simulink model "lab4_sim"  (R2022b)
settings: Solver=VariableStepAuto  StartTime=0.0  StopTime=10.0  RelTol=1e-3
values from neighbouring files (symbols this model uses):
  A = [0 0 1 0; 0 0 0 1; -(k1 + k2)/m1 k2/m1 -(c1 + c2)/m1 c2/m1; k2/m2 -k2/m2 c2/m2 -c2/m2]    [lab4.m]    (also in test.m)
  B = [(c1/m1) 0 0; 0 0 0; (k1/m1) - ((c1 + c2)*c1)/(m1*m1) (k1 + k2)/m1 k2/m1 ; (c1*c2)/(m1*m2) k2/m2 -k2/m2]    [lab4.m]    (also in test.m = [(c1/m1); 0; (k1/m1) - ((c1 + c2)*c1)/(m1*m1); (c1*c2)/(m1*m)
  C = [1 0 0 0; 0 1 0 0; 0 0 1 0; 0 0 0 1]    [lab4.m]    (also in test.m = eye(4,4))
  c1 = 100    [lab4.m]    (also in test.m)
  c2 = 2000    [lab4.m]    (also in test.m)
  D = [0 0 0; 0 0 0; 0 0 0; 0 0 0]    [lab4.m]    (also in test.m = [0; 0; 0; 0])
  k1 = 370000    [lab4.m]    (also in test.m)
  k2 = 35000    [lab4.m]    (also in test.m)
  m1 = 90    [lab4.m]    (also in test.m)
  m2 = 600    [lab4.m]    (also in test.m)
  x10 = 0.2    [lab4.m]
  x20 = 1    [lab4.m]
settings Model: Creator=karol  LastModifiedBy=karol

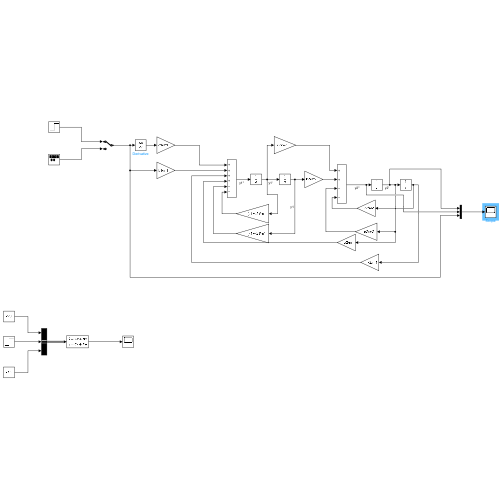
[thumbnail: Simulink's stored preview of the top-level diagram]
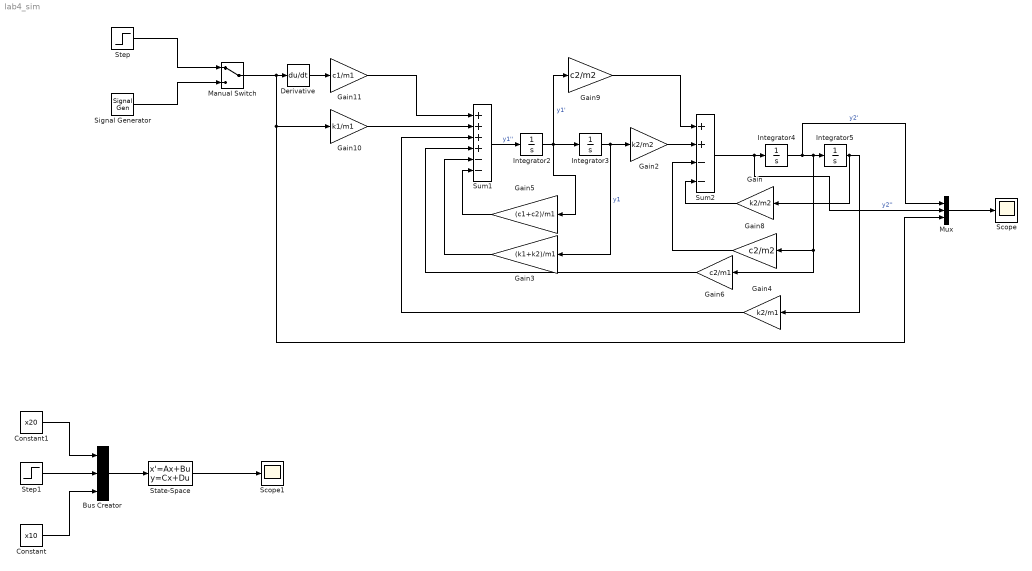
== system lab4_sim ==
  Bus Creator : BusCreator  Inputs=3
  Constant : Constant  Value=x10
  Constant1 : Constant  Value=x20
  Derivative : Derivative
  Gain : Gain  Gain=k2/m2
  Gain10 : Gain  Gain=k1/m1
  Gain11 : Gain  Gain=c1/m1
  Gain2 : Gain  Gain=k2/m2
  Gain3 : Gain  Gain=(k1+k2)/m1
  Gain4 : Gain  Gain=k2/m1
  Gain5 : Gain  Gain=(c1+c2)/m1
  Gain6 : Gain  Gain=c2/m1
  Gain8 : Gain  Gain=c2/m2
  Gain9 : Gain  Gain=c2/m2
  Integrator{2..5} (4 alike) : Integrator
  Manual Switch : ManualSwitch
  Mux : Mux  Inputs=3
  Scope : Scope
  Scope1 : Scope
  Signal Generator : SignalGenerator  WaveForm=sawtooth  Amplitude=0.1  Units=rad/sec
  State-Space : StateSpace  A=A  B=B  C=C  D=D  InitialCondition=0
  Step : Step  After=0.1  SampleTime=0
  Step1 : Step  After=0.1  SampleTime=0
  Sum1 : Sum  Inputs=++++--
  Sum2 : Sum  Inputs=++--
  wires:
  Sum1/1 -> Integrator2/1  "y1''"
  Integrator2/1 -> Gain5/1, Integrator3/1, Gain9/1  "y1'"
  Integrator3/1 -> Gain3/1, Gain2/1  "y1"
  Gain2/1 -> Sum2/2
  Sum2/1 -> Mux/2, Integrator4/1  "y2''"
  Integrator4/1 -> Mux/1, Gain6/1, Gain8/1, Integrator5/1  "y2'"
  Gain3/1 -> Sum1/5
  Step/1 -> Manual Switch/1
  Integrator5/1 -> Gain/1, Gain4/1
  Gain4/1 -> Sum1/3
  Gain5/1 -> Sum1/6
  Gain6/1 -> Sum1/4
  Gain8/1 -> Sum2/3
  Gain9/1 -> Sum2/1
  Gain10/1 -> Sum1/2
  Derivative/1 -> Gain11/1
  Gain11/1 -> Sum1/1
  Mux/1 -> Scope/1
  Manual Switch/1 -> Mux/3, Gain10/1, Derivative/1
  Signal Generator/1 -> Manual Switch/2
  Gain/1 -> Sum2/4
  State-Space/1 -> Scope1/1
  Step1/1 -> Bus Creator/2
  Bus Creator/1 -> State-Space/1
  Constant1/1 -> Bus Creator/1
  Constant/1 -> Bus Creator/3
